simulink model "pendolo_2integratori"  (R2020b)
settings: Solver=VariableStepAuto  StartTime=0.0  StopTime=20  RelTol=1e-3
values from neighbouring files (symbols this model uses):
  a = 0.25    [finvpend.m]    (also in pendolo_inverso.m)
  g = 9.81    [equilibrio.m]    (also in finvpend.m; pendolo_inverso.m)
  k = 4.5    [equilibrio.m]    (also in finvpend.m; pendolo_inverso.m)
  L = 0.5    [equilibrio.m]    (also in finvpend.m; pendolo_inverso.m)
  m = 1    [equilibrio.m]    (also in finvpend.m; pendolo_inverso.m)
settings Model: Creator=Lenovo  LastModifiedBy=Lenovo

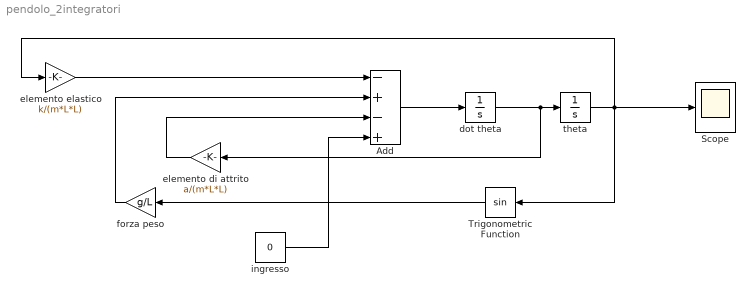
== system pendolo_2integratori ==
  Add : Sum  Inputs=-+-+
  Scope : Scope
  Trigonometric Function : Trigonometry
  dot theta : Integrator
  elemento di attrito : Gain  Gain=a/(m*L*L)
  elemento elastico : Gain  Gain=k/(m*L*L)
  forza peso : Gain  Gain=g/L
  ingresso : Constant  Value=0
  theta : Integrator  InitialCondition=0.7
  wires:
  dot theta/1 -> elemento di attrito/1, theta/1
  theta/1 -> Scope/1, Trigonometric Function/1, elemento elastico/1
  Add/1 -> dot theta/1
  Trigonometric Function/1 -> forza peso/1
  forza peso/1 -> Add/2
  elemento elastico/1 -> Add/1
  elemento di attrito/1 -> Add/3
  ingresso/1 -> Add/4
